simulink subsystem "unitcell"  (R2022b)
settings: Solver=VariableStepAuto  StartTime=0.0  StopTime=10.0  RelTol=1e-3
libraries: dspsigops x4
settings Model: Creator=padlewsk  LastModifiedBy=padlewsk

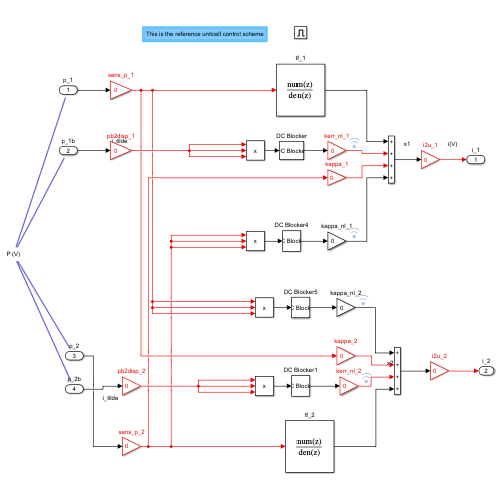
[thumbnail: Simulink's stored preview of the top-level diagram]
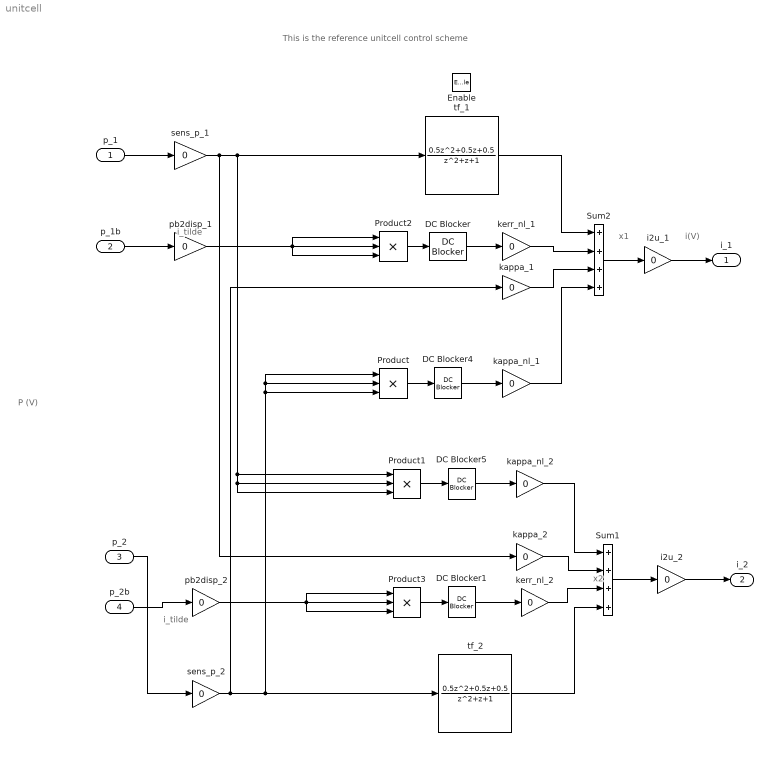
== system unitcell ==
  note: This is the reference unitcell control scheme
  note: x2
  note: P (V)
  note: i_tilde
  note: i(V)
  note: i_tilde
  note: x1
  p_1 : Inport
  p_1b : Inport  Port=2
  p_2 : Inport  Port=3
  p_2b : Inport  Port=4
  Enable : EnablePort
  DC Blocker{,1,4..5} (4 alike) : dspsigops/DC Blocker  Algorithm=FIR  NormalizedBandwidth=0.001  Length=50  Order=6  SimulateUsing=Code generation
      settings: LibrarySourceBlock=dsphdlsupportsigops/DC Blocker
  Product{,1..3} (4 alike) : Product  Inputs=3
  Sum1 : Sum  Inputs=++++
  Sum2 : Sum  Inputs=++++
  i2u_1 : Gain  Gain=0
  i2u_2 : Gain  Gain=0
  kappa_1 : Gain  Gain=0
  kappa_2 : Gain  Gain=0
  kappa_nl_1 : Gain  Gain=0
  kappa_nl_2 : Gain  Gain=0
  kerr_nl_1 : Gain  Gain=0
  kerr_nl_2 : Gain  Gain=0
  pb2disp_1 : Gain  Gain=0
  pb2disp_2 : Gain  Gain=0
  sens_p_1 : Gain  Gain=0
  sens_p_2 : Gain  Gain=0
  tf_1 : DiscreteTransferFcn  Numerator="[0.5         0.5         0.5]"  Denominator="[1  1  1]"
  tf_2 : DiscreteTransferFcn  Numerator="[0.5         0.5         0.5]"  Denominator="[1  1  1]"
  i_1 : Outport
  i_2 : Outport  Port=2
  wires:
  p_2/1 -> sens_p_2/1
  p_2b/1 -> pb2disp_2/1
  p_1/1 -> sens_p_1/1
  i2u_1/1 -> i_1/1
  i2u_2/1 -> i_2/1
  kerr_nl_2/1 -> Sum1/3
  tf_2/1 -> Sum1/4
  Sum1/1 -> i2u_2/1
  kerr_nl_1/1 -> Sum2/2
  tf_1/1 -> Sum2/1
  Sum2/1 -> i2u_1/1
  Product3/1 -> DC Blocker1/1
  Product2/1 -> DC Blocker/1
  DC Blocker/1 -> kerr_nl_1/1
  DC Blocker1/1 -> kerr_nl_2/1
  p_1b/1 -> pb2disp_1/1
  sens_p_1/1 -> kappa_2/1, tf_1/1, Product1/1, Product1/2, Product1/3
  sens_p_2/1 -> kappa_1/1, tf_2/1, Product/3, Product/1, Product/2
  kappa_1/1 -> Sum2/3
  kappa_2/1 -> Sum1/2
  Product1/1 -> DC Blocker5/1
  DC Blocker4/1 -> kappa_nl_1/1
  kappa_nl_1/1 -> Sum2/4
  DC Blocker5/1 -> kappa_nl_2/1
  kappa_nl_2/1 -> Sum1/1
  Product/1 -> DC Blocker4/1
  pb2disp_2/1 -> Product3/3, Product3/2, Product3/1
  pb2disp_1/1 -> Product2/2, Product2/3, Product2/1
